simulink model "open_loop_dyn"  (R2022a)
settings: Solver=VariableStepAuto  StartTime=0.0  StopTime=10.0  RelTol=1e-3
undefined symbols (not defined in the file or in its folder): f0, n0, tau_qm
settings Model: Creator=charl  LastModifiedBy=charl

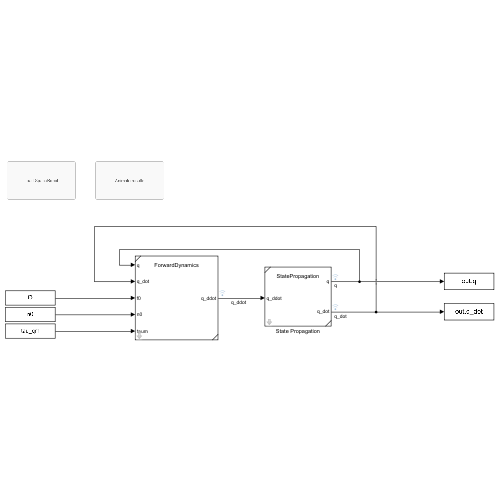
[thumbnail: Simulink's stored preview of the top-level diagram]
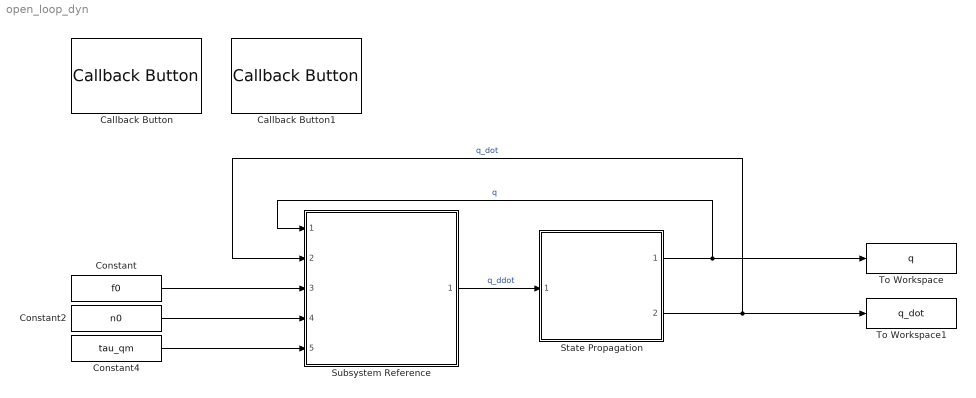
== system open_loop_dyn ==
  Callback Button : CallbackButton  ButtonText=Load SpaceRobot
      settings: ClickFcn=|
      | load('SC_2DoF.mat')
      | sc.homeConfig;
  Callback Button1 : CallbackButton  ButtonText=Animate results
      settings: ClickFcn=|
      | close all
      | dim = [.2 .5 .3 .3];
      | 
      | framesPerSecond = length(simRes.tout)/simRes.tout(end);
      | r = rateControl(framesPerSecond);
      | str = sprintf('t = %.2fs', 0);
      | h_annot = annotation('textbox', dim,'String', str,'FitBoxToText','on');
      | 
      | for i = 1:length(simRes.q.Time)
      |     sc.q = simRes.q.Data(:, :, i);
      |     sc.show('preserve', false, 'fast', true, 'visuals', 'on');
      |     curT = i/framesPerSecond;
      |     str = sprintf('t = %.2fs', curT);
      |     h_annot.set('String',str);
      |     drawnow
      | %     waitfor(r);
      | end
      | close all
  Constant : Constant  Value=f0
  Constant2 : Constant  Value=n0
  Constant4 : Constant  Value=tau_qm
  State Propagation : Subsystem  ReferencedSubsystem=StatePropagation  spaceRobot=sc
  Subsystem Reference : Subsystem  ReferencedSubsystem=ForwardDynamics  spaceRobot=sc  SimulateUsing=Interpreted execution
  To Workspace : ToWorkspace  VariableName=q  SaveFormat=Timeseries  SampleTime=-1
  To Workspace1 : ToWorkspace  VariableName=q_dot  SaveFormat=Timeseries  SampleTime=-1
  wires:
  Subsystem Reference/1 -> State Propagation/1  "q_ddot"
  Constant4/1 -> Subsystem Reference/5
  Constant2/1 -> Subsystem Reference/4
  State Propagation/1 -> Subsystem Reference/1, To Workspace/1  "q"
  State Propagation/2 -> Subsystem Reference/2, To Workspace1/1  "q_dot"
  Constant/1 -> Subsystem Reference/3
